simulink model "sl_subsys_fcncallerr7"  (Simulink 6.0)
settings: Solver=FixedStepDiscrete  StartTime=0.0  StopTime=10.0  FixedStep=1  RelTol=1e-3
settings Model: CovMetricSettings=d  Creator=The MathWorks Inc.  LastModifiedBy=batserve  ExtModeAutoUpdateStatusClock=off
settings OptimizationCC: BlockReduction=off  BooleanDataType=off
settings DebuggingCC: CheckExecutionContextPreStartOutputMsg=on  CheckExecutionContextRuntimeOutputMsg=on  SolverPrmCheckMsg=none
settings HardwareCC: TargetUnknown=on

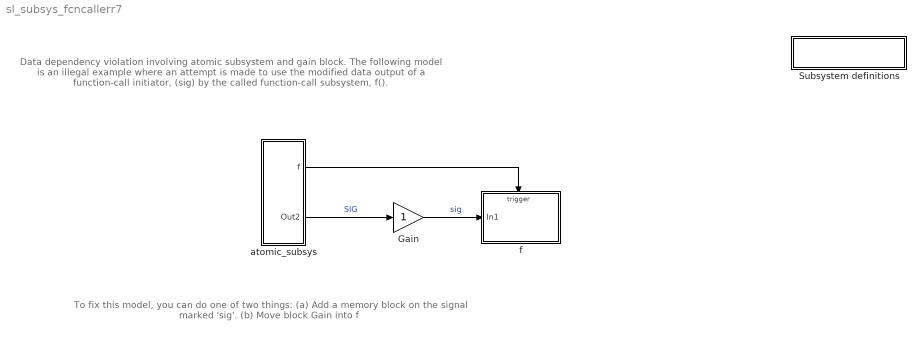
== system sl_subsys_fcncallerr7 ==
  note: To fix this model, you can do one of two things:
      | (a) Add a memory block on the signal marked 'sig'.
      | (b) Move block Gain into f
  note: Data dependency violation involving atomic subsystem and gain block.
      |
      | The following model is an illegal example where an attempt is made
      | to use the modified data output of a function-call initiator, (sig)
      | by the called function-call subsystem, f().
  " Subsystem definitions" : Subsystem  PropExecContextAcrossSSBoundary=on
      settings: OpenFcn=helpview([matlabroot,'/toolbox/simulink/simdemos/sl_subsys_definitions.html']);
      mask Display: disp('Subsystem\ndefinitions')
  Gain : Gain  SaturateOnIntegerOverflow=on
  atomic_subsys : Subsystem  TreatAsAtomicUnit=on  PropExecContextAcrossSSBoundary=on
  f : Subsystem  TreatAsAtomicUnit=on  PropExecContextAcrossSSBoundary=on
  wires:
  atomic_subsys/2(Out2) -> Gain/1  "SIG"
  atomic_subsys/1(f) -> f/Trigger
  Gain/1 -> f/1(In1)  "sig"

== system sl_subsys_fcncallerr7/ Subsystem definitions ==

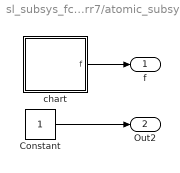
== system sl_subsys_fcncallerr7/atomic_subsys ==
  Constant : Constant
  chart : Stateflow chart  PropExecContextAcrossSSBoundary=on
  f : Outport
  Out2 : Outport  Port=2
  wires:
  Constant/1 -> Out2/1
  chart/1(f) -> f/1

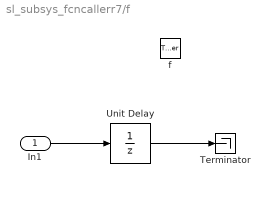
== system sl_subsys_fcncallerr7/f ==
  In1 : Inport  Port=1  LatchInput=off
  f : TriggerPort  TriggerType=function-call
  Terminator : Terminator
  Unit Delay : UnitDelay  SampleTime=-1
  wires:
  In1/1 -> Unit Delay/1
  Unit Delay/1 -> Terminator/1

== stateflow chart atomic_subsys/chart ==
  state one/
    entry: f;
  state two/
    entry: f;
  one -> two
  two -> one
  (default) -> one
  events: f output FUNCTION_CALL_EVENT
